simulink model "mimo2"  (R2021b)
settings: Solver=VariableStepAuto  StartTime=0.0  StopTime=500  RelTol=1e-3
libraries: cstblocks x3
settings Model: Creator=Hu  LastModifiedBy=Hu

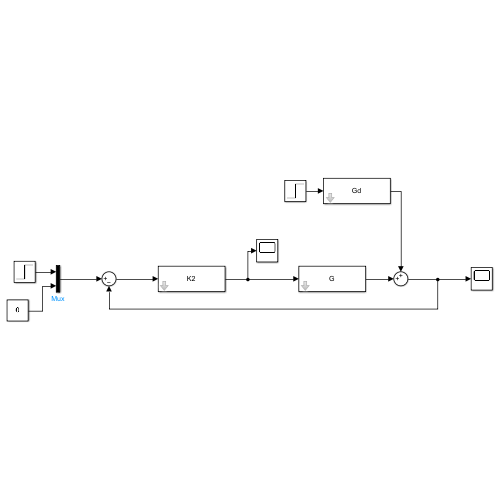
[thumbnail: Simulink's stored preview of the top-level diagram]
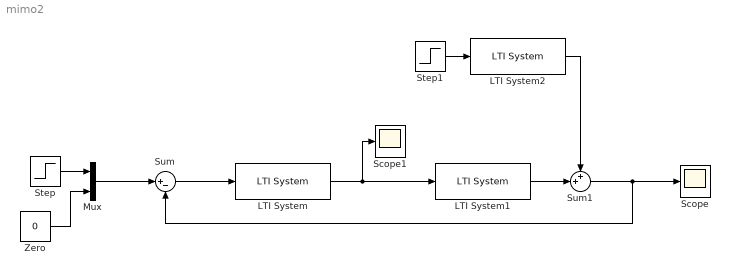
== system mimo2 ==
  LTI System : cstblocks/LTI System  sys=K2  IC=[]
  LTI System1 : cstblocks/LTI System  sys=G  IC=[]
  LTI System2 : cstblocks/LTI System  sys=Gd  IC=[]
  Mux : Mux  Inputs=2
  Scope : Scope
  Scope1 : Scope
  Step : Step  SampleTime=0
  Step1 : Step  SampleTime=0
  Sum : Sum  Inputs=|+-
  Sum1 : Sum  Inputs=++|
  Zero : Constant  Value=0  OutDataTypeStr=Inherit: Inherit via back propagation
  wires:
  Step/1 -> Mux/1
  Zero/1 -> Mux/2
  LTI System/1 -> Scope1/1, LTI System1/1
  Mux/1 -> Sum/1
  Sum/1 -> LTI System/1
  Step1/1 -> LTI System2/1
  LTI System1/1 -> Sum1/2
  Sum1/1 -> Sum/2, Scope/1
  LTI System2/1 -> Sum1/1
